simulink model "conservative"  (R2016a)
settings: Solver=VariableStepAuto  StartTime=0.0  StopTime=2  MaxStep=0.002  MinStep=0.001  RelTol=1e-3
settings Model: Creator=Jann dan Jursus  LastModifiedBy=Jann dan Jursus
settings SolverCC: InitialStep=0.001

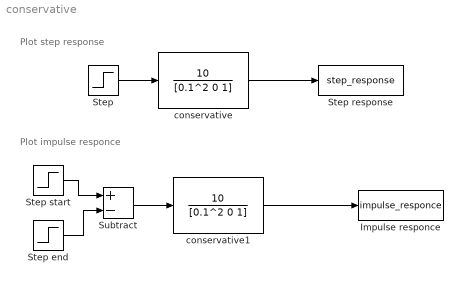
== system conservative ==
  note: Plot impulse responce
  note: Plot step response
  Impulse responce : ToWorkspace  VariableName=impulse_responce  SaveFormat=Timeseries  SampleTime=-1
  Step : Step  Time=0  SampleTime=0
  Step end : Step  Time=1.001  After=100  SampleTime=0
  Step response : ToWorkspace  VariableName=step_response  SaveFormat=Timeseries  SampleTime=-1
  Step start : Step  After=100  SampleTime=0
  Subtract : Sum  Inputs=+-
  conservative : TransferFcn  Numerator=[10]  Denominator=[0.1^2 0 1]
  conservative1 : TransferFcn  Numerator=[10]  Denominator=[0.1^2 0 1]
  wires:
  Step start/1 -> Subtract/1
  Step end/1 -> Subtract/2
  Subtract/1 -> conservative1/1
  Step/1 -> conservative/1
  conservative/1 -> Step response/1
  conservative1/1 -> Impulse responce/1
